simulink model "model_grad_wl"  (R2022a)
settings: Solver=VariableStepAuto  StartTime=0.0  StopTime=1000  MaxStep=1e-3  RelTol=1e-3
values from neighbouring files (symbols this model uses):
  b_m = b_0    (= 7)    [config.m]
  gamma_grad = 100000000    [task_grad.m]    (also in tasks.m)
  k_0 = 1    [config.m]
  K_M = K_M_g    [config.m]
  Lambda = -k_0    (= -1)    [config.m]
  nu1 = zeros(length(Lambda), 1)    [config.m]
  nu2 = zeros(length(Lambda), 1)    [config.m]
  object_denum = [1 a_1 a_0]    [config.m]
  object_num = [b_0]    [config.m]
  psi_hat_init_conds = zeros(omega_size, 1)    [config.m]
settings Model: SimulationMode=accelerator  LastModifiedBy=Vvlad
settings OptimizationCC: BlockReduction=off  BooleanDataType=off
settings DebuggingCC: SaveWithParameterizedLinksMsg=none  UnderspecifiedInitializationDetection=Classic  MergeDetectMultiDrivingBlocksExec=none  SignalResolutionControl=TryResolveAllWithWarning  UnconnectedInputMsg=warning  UnconnectedOutputMsg=warning  UnconnectedLineMsg=warning
settings HardwareCC: TargetUnknown=on
settings ModelReferenceCC: PropagateSignalLabelsOutOfModel=off
settings RTWCC: DLArmComputeVersion=19.05

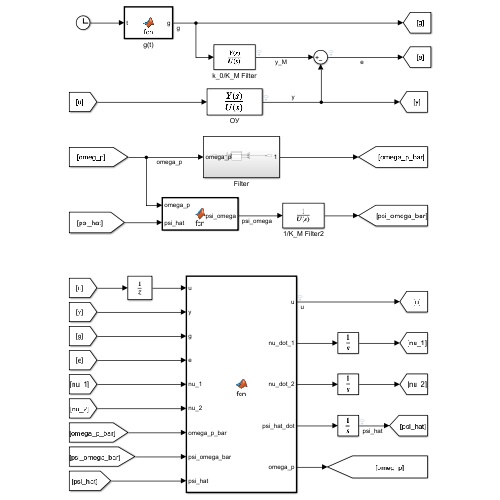
[thumbnail: Simulink's stored preview of the top-level diagram]
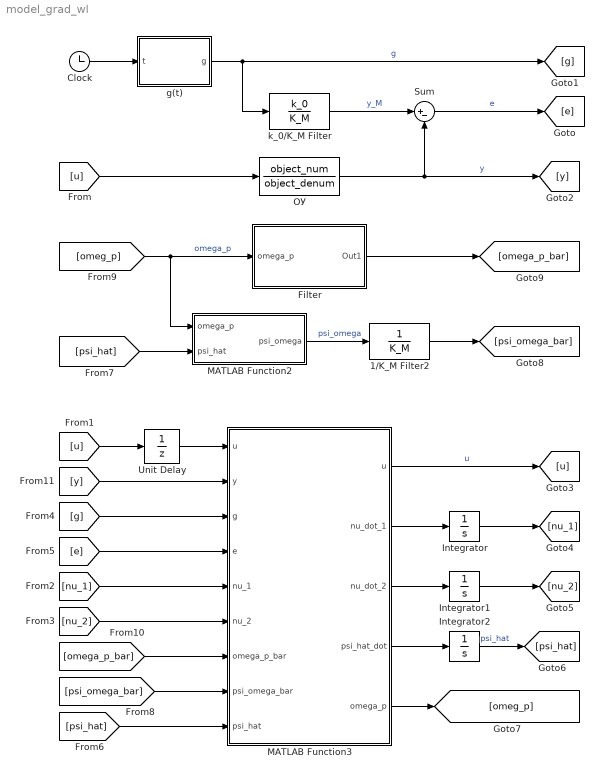
== system model_grad_wl ==
  1/K_M Filter2 : TransferFcn  Denominator=K_M
  Clock : Clock
  Filter : Subsystem
  Integrator : Integrator  InitialCondition=nu1
  Integrator1 : Integrator  InitialCondition=nu2
  Integrator2 : Integrator  InitialCondition=psi_hat_init_conds
  MATLAB Function2 : MATLAB Function  TreatAsAtomicUnit=on
  MATLAB Function3 : MATLAB Function  TreatAsAtomicUnit=on
  Sum : Sum  Inputs=|+-
  Unit Delay : UnitDelay  SampleTime=-1  HasFrameUpgradeWarning=on
  g(t) : MATLAB Function  TreatAsAtomicUnit=on
  k_0/K_M Filter : TransferFcn  Numerator=k_0  Denominator=K_M
  ОУ : TransferFcn  Numerator=object_num  Denominator=object_denum
  wires:
  [omeg_p] -> Filter/1(omega_p), MATLAB Function2/1(omega_p)  "omega_p"
  1/K_M Filter2/1 -> [psi_omega_bar]
  MATLAB Function2/1(psi_omega) -> 1/K_M Filter2/1  "psi_omega"
  Filter/1(Out1) -> [omega_p_bar]
  [u] -> ОУ/1
  k_0/K_M Filter/1 -> Sum/1  "y_M"
  Sum/1 -> [e]  "e"
  ОУ/1 -> [y], Sum/2  "y"
  g(t)/1(g) -> [g], k_0/K_M Filter/1  "g"
  Clock/1 -> g(t)/1(t)
  MATLAB Function3/1(u) -> [u]  "u"
  [u] -> Unit Delay/1
  Unit Delay/1 -> MATLAB Function3/1("u ")
  MATLAB Function3/3(nu_dot_2) -> Integrator1/1
  MATLAB Function3/2(nu_dot_1) -> Integrator/1
  Integrator/1 -> [nu_1]
  Integrator1/1 -> [nu_2]
  [nu_1] -> MATLAB Function3/5(nu_1)
  [nu_2] -> MATLAB Function3/6(nu_2)
  [e] -> MATLAB Function3/4(e)
  [g] -> MATLAB Function3/3(g)
  MATLAB Function3/4(psi_hat_dot) -> Integrator2/1
  Integrator2/1 -> [psi_hat]  "psi_hat"
  [psi_hat] -> MATLAB Function3/9(psi_hat)
  [psi_hat] -> MATLAB Function2/2(psi_hat)
  MATLAB Function3/5(omega_p) -> [omeg_p]
  [psi_omega_bar] -> MATLAB Function3/8(psi_omega_bar)
  [omega_p_bar] -> MATLAB Function3/7(omega_p_bar)
  [y] -> MATLAB Function3/2(y)

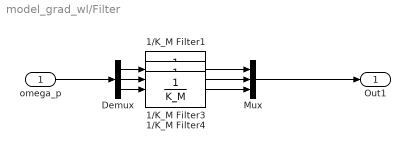
== system model_grad_wl/Filter ==
  omega_p : Inport
  1/K_M Filter1 : TransferFcn  Denominator=K_M
  1/K_M Filter3 : TransferFcn  Denominator=K_M
  1/K_M Filter4 : TransferFcn  Denominator=K_M
  Demux : Demux  Outputs=3
  Mux : Mux  Inputs=3
  Out1 : Outport
  wires:
  1/K_M Filter1/1 -> Mux/1
  Demux/2 -> 1/K_M Filter3/1
  Demux/3 -> 1/K_M Filter4/1
  1/K_M Filter4/1 -> Mux/3
  Mux/1 -> Out1/1
  1/K_M Filter3/1 -> Mux/2
  Demux/1 -> 1/K_M Filter1/1
  omega_p/1 -> Demux/1

== matlab function model_grad_wl/g(t) ==
  data: t input; g output
function g = fcn(t)

g = 7*sin(8*t+1);

== matlab function model_grad_wl/MATLAB Function2 ==
  data: omega_p input; psi_hat input; psi_omega output
function psi_omega = fcn(omega_p, psi_hat)
 psi_omega = psi_hat'*omega_p;

== matlab function model_grad_wl/MATLAB Function3 ==
  data: u input; y input; g input; e input; nu_1 input; nu_2 input; u output; nu_dot_1 output; nu_dot_2 output; omega_p_bar input; psi_hat_dot output; omega_p output; psi_omega_bar input; psi_hat input; Lambda parameter; b_m parameter; k_0 parameter; gamma_grad parameter
function [u, nu_dot_1, nu_dot_2, psi_hat_dot, omega_p] = fcn(u, y, g, e, nu_1, nu_2, omega_p_bar, psi_omega_bar, psi_hat, Lambda, b_m, k_0, gamma_grad)

nu_dot_1 = Lambda*nu_1 + u;
nu_dot_2 = Lambda*nu_2 + y;
omega = [nu_1', nu_2', y]';
omega_p = -omega;

e_hat = e - psi_hat'*omega_p_bar + psi_omega_bar;
psi_hat_dot = gamma_grad*omega_p_bar*e_hat/(1+omega_p_bar'*omega_p_bar);
u = (psi_hat'*omega_p+k_0*g)/b_m;
